simulink model "nn"  (R2018b)
settings: Solver=VariableStepAuto  StartTime=0.0  StopTime=10.0  RelTol=1e-3
libraries: neural x28
settings Model: Creator=Mihail  LastModifiedBy=Mihail

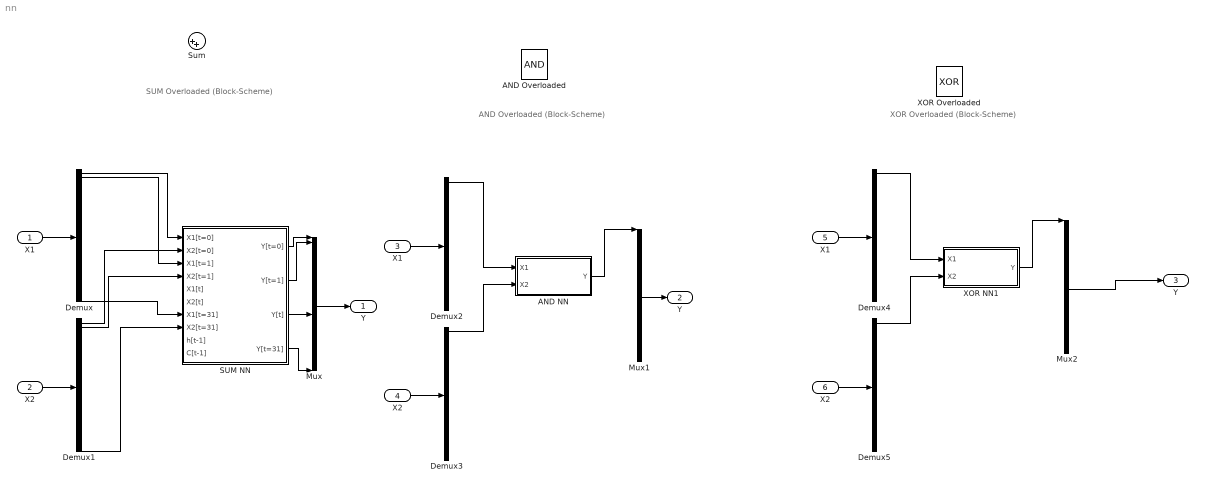
== system nn ==
  note: SUM Overloaded
      | (Block-Scheme)
  note: AND Overloaded
      | (Block-Scheme)
  note: XOR Overloaded
      | (Block-Scheme)
  X1 : Inport
  X2 : Inport  Port=2
  "X1 " : Inport  Port=3
  "X2 " : Inport  Port=4
  "X1   " : Inport  Port=5
  "X2  " : Inport  Port=6
  AND NN : Subsystem
  AND Overloaded : Logic  AllPortsSameDT=off  OutDataTypeStr=boolean
  Demux{,1..5} (6 alike) : Demux  Outputs=32
  Mux : Mux  Inputs=32
  Mux1 : Mux  Inputs=32
  Mux2 : Mux  Inputs=32
  SUM NN : Subsystem
  Sum : Sum  Inputs=|++
  XOR NN1 : Subsystem
  XOR Overloaded : Logic  Operator=XOR  AllPortsSameDT=off  OutDataTypeStr=boolean
  Y : Outport
  "Y " : Outport  Port=2
  "Y  " : Outport  Port=3
  wires:
  Demux/2 -> SUM NN/1(X1[t=0])
  Demux1/2 -> SUM NN/2(X2[t=0])
  Demux/3 -> SUM NN/3(X1[t=1])
  SUM NN/1(Y[t=0]) -> Mux/1
  SUM NN/2(Y[t=1]) -> Mux/2
  SUM NN/3(Y[t]) -> Mux/19
  SUM NN/4(Y[t=31]) -> Mux/32
  Demux/32 -> SUM NN/7(X1[t=31])
  Demux1/3 -> SUM NN/4(X2[t=1])
  Demux1/32 -> SUM NN/8(X2[t=31])
  X1/1 -> Demux/1
  X2/1 -> Demux1/1
  Mux/1 -> Y/1
  AND NN/1(Y) -> Mux1/1
  "X1 "/1 -> Demux2/1
  "X2 "/1 -> Demux3/1
  Demux2/2 -> AND NN/1(X1)
  Demux3/2 -> AND NN/2(X2)
  Mux1/1 -> "Y "/1
  Demux4/2 -> XOR NN1/1(X1)
  "X1   "/1 -> Demux4/1
  "X2  "/1 -> Demux5/1
  Demux5/2 -> XOR NN1/2(X2)
  XOR NN1/1(Y) -> Mux2/1
  Mux2/1 -> "Y  "/1

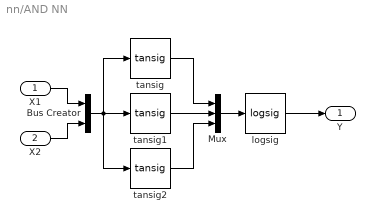
== system nn/AND NN ==
  X1 : Inport
  X2 : Inport  Port=2
  Bus Creator : BusCreator  Inputs=2
  Mux : Mux  Inputs=3
  logsig : neural/Transfer Functions/logsig
  tansig : neural/Transfer Functions/tansig
  tansig1 : neural/Transfer Functions/tansig
  tansig2 : neural/Transfer Functions/tansig
  Y : Outport
  wires:
  tansig2/1 -> Mux/3
  tansig1/1 -> Mux/2
  tansig/1 -> Mux/1
  Mux/1 -> logsig/1
  logsig/1 -> Y/1
  X1/1 -> Bus Creator/1
  X2/1 -> Bus Creator/2
  Bus Creator/1 -> tansig/1, tansig2/1, tansig1/1

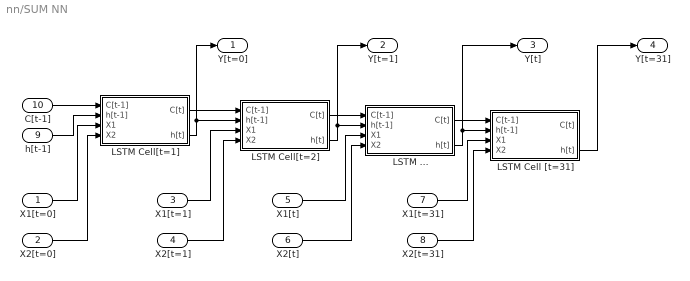
== system nn/SUM NN ==
  X1[t=0] : Inport
  X2[t=0] : Inport  Port=2
  X1[t=1] : Inport  Port=3
  X2[t=1] : Inport  Port=4
  X1[t] : Inport  Port=5
  X2[t] : Inport  Port=6
  X1[t=31] : Inport  Port=7
  X2[t=31] : Inport  Port=8
  h[t-1] : Inport  Port=9
  C[t-1] : Inport  Port=10
  LSTM ... : Subsystem
  LSTM Cell [t=31] : Subsystem
  LSTM Cell[t=1] : Subsystem
  LSTM Cell[t=2] : Subsystem
  Y[t=0] : Outport
  Y[t=1] : Outport  Port=2
  Y[t] : Outport  Port=3
  Y[t=31] : Outport  Port=4
  wires:
  C[t-1]/1 -> LSTM Cell[t=1]/1(C[t-1])
  h[t-1]/1 -> LSTM Cell[t=1]/2(h[t-1])
  LSTM Cell[t=1]/1(C[t]) -> LSTM Cell[t=2]/1(C[t-1])
  LSTM Cell[t=1]/2(h[t]) -> Y[t=0]/1, LSTM Cell[t=2]/2(h[t-1])
  X1[t=0]/1 -> LSTM Cell[t=1]/3(X1)
  X2[t=0]/1 -> LSTM Cell[t=1]/4(X2)
  X1[t=1]/1 -> LSTM Cell[t=2]/3(X1)
  X2[t=1]/1 -> LSTM Cell[t=2]/4(X2)
  LSTM Cell[t=2]/1(C[t]) -> LSTM .../1(C[t-1])
  LSTM Cell[t=2]/2(h[t]) -> Y[t=1]/1, LSTM .../2(h[t-1])
  LSTM .../1(C[t]) -> LSTM Cell [t=31]/1(C[t-1])
  X2[t]/1 -> LSTM .../4(X2)
  X1[t]/1 -> LSTM .../3(X1)
  X1[t=31]/1 -> LSTM Cell [t=31]/3(X1)
  X2[t=31]/1 -> LSTM Cell [t=31]/4(X2)
  LSTM Cell [t=31]/2(h[t]) -> Y[t=31]/1
  LSTM .../2(h[t]) -> Y[t]/1, LSTM Cell [t=31]/2(h[t-1])

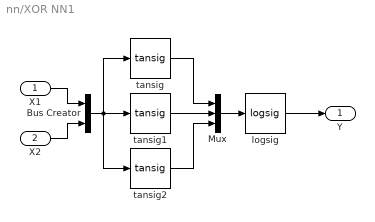
== system nn/XOR NN1 ==
  X1 : Inport
  X2 : Inport  Port=2
  Bus Creator : BusCreator  Inputs=2
  Mux : Mux  Inputs=3
  logsig : neural/Transfer Functions/logsig
  tansig : neural/Transfer Functions/tansig
  tansig1 : neural/Transfer Functions/tansig
  tansig2 : neural/Transfer Functions/tansig
  Y : Outport
  wires:
  tansig2/1 -> Mux/3
  tansig1/1 -> Mux/2
  tansig/1 -> Mux/1
  Mux/1 -> logsig/1
  logsig/1 -> Y/1
  X1/1 -> Bus Creator/1
  X2/1 -> Bus Creator/2
  Bus Creator/1 -> tansig/1, tansig2/1, tansig1/1

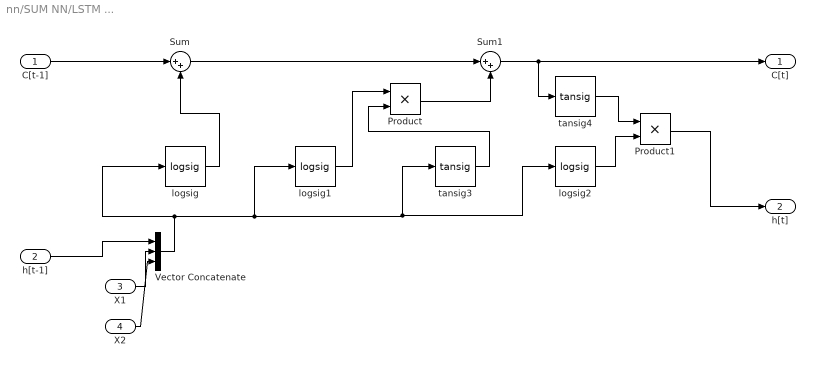
== system nn/SUM NN/LSTM ... ==
  C[t-1] : Inport
  h[t-1] : Inport  Port=2
  X1 : Inport  Port=3
  X2 : Inport  Port=4
  Product : Product
  Product1 : Product
  Sum : Sum  Inputs=|++
  Sum1 : Sum  Inputs=|++
  Vector Concatenate : Concatenate  NumInputs=3
  logsig : neural/Transfer Functions/logsig
  logsig1 : neural/Transfer Functions/logsig
  logsig2 : neural/Transfer Functions/logsig
  tansig3 : neural/Transfer Functions/tansig
  tansig4 : neural/Transfer Functions/tansig
  C[t] : Outport
  h[t] : Outport  Port=2
  wires:
  h[t-1]/1 -> Vector Concatenate/1
  X1/1 -> Vector Concatenate/2
  X2/1 -> Vector Concatenate/3
  Vector Concatenate/1 -> tansig3/1, logsig2/1, logsig1/1, logsig/1
  C[t-1]/1 -> Sum/1
  logsig/1 -> Sum/2
  Sum/1 -> Sum1/1
  tansig3/1 -> Product/2
  logsig1/1 -> Product/1
  Product/1 -> Sum1/2
  logsig2/1 -> Product1/2
  Sum1/1 -> C[t]/1, tansig4/1
  tansig4/1 -> Product1/1
  Product1/1 -> h[t]/1

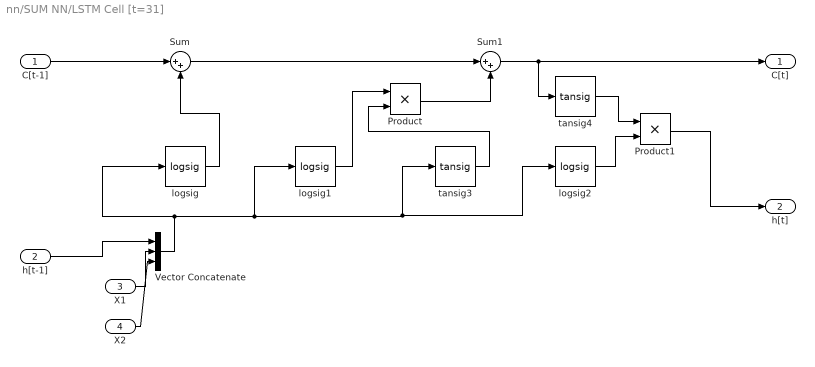
== system nn/SUM NN/LSTM Cell [t=31] ==
  C[t-1] : Inport
  h[t-1] : Inport  Port=2
  X1 : Inport  Port=3
  X2 : Inport  Port=4
  Product : Product
  Product1 : Product
  Sum : Sum  Inputs=|++
  Sum1 : Sum  Inputs=|++
  Vector Concatenate : Concatenate  NumInputs=3
  logsig : neural/Transfer Functions/logsig
  logsig1 : neural/Transfer Functions/logsig
  logsig2 : neural/Transfer Functions/logsig
  tansig3 : neural/Transfer Functions/tansig
  tansig4 : neural/Transfer Functions/tansig
  C[t] : Outport
  h[t] : Outport  Port=2
  wires:
  h[t-1]/1 -> Vector Concatenate/1
  X1/1 -> Vector Concatenate/2
  X2/1 -> Vector Concatenate/3
  Vector Concatenate/1 -> tansig3/1, logsig2/1, logsig1/1, logsig/1
  C[t-1]/1 -> Sum/1
  logsig/1 -> Sum/2
  Sum/1 -> Sum1/1
  tansig3/1 -> Product/2
  logsig1/1 -> Product/1
  Product/1 -> Sum1/2
  logsig2/1 -> Product1/2
  Sum1/1 -> C[t]/1, tansig4/1
  tansig4/1 -> Product1/1
  Product1/1 -> h[t]/1

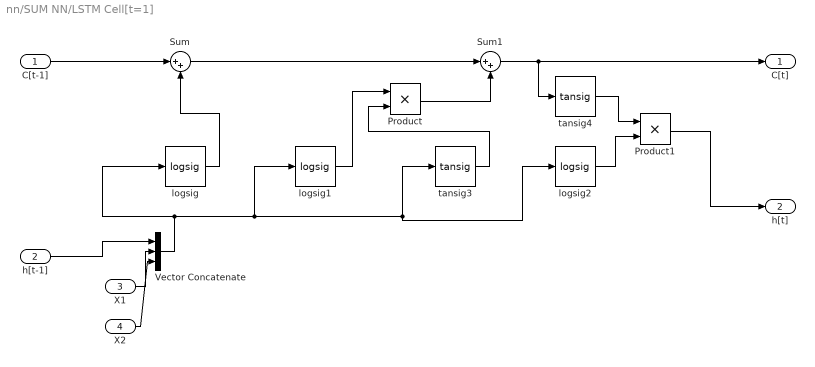
== system nn/SUM NN/LSTM Cell[t=1] ==
  C[t-1] : Inport
  h[t-1] : Inport  Port=2
  X1 : Inport  Port=3
  X2 : Inport  Port=4
  Product : Product
  Product1 : Product
  Sum : Sum  Inputs=|++
  Sum1 : Sum  Inputs=|++
  Vector Concatenate : Concatenate  NumInputs=3
  logsig : neural/Transfer Functions/logsig
  logsig1 : neural/Transfer Functions/logsig
  logsig2 : neural/Transfer Functions/logsig
  tansig3 : neural/Transfer Functions/tansig
  tansig4 : neural/Transfer Functions/tansig
  C[t] : Outport
  h[t] : Outport  Port=2
  wires:
  h[t-1]/1 -> Vector Concatenate/1
  X1/1 -> Vector Concatenate/2
  X2/1 -> Vector Concatenate/3
  Vector Concatenate/1 -> tansig3/1, logsig2/1, logsig1/1, logsig/1
  C[t-1]/1 -> Sum/1
  logsig/1 -> Sum/2
  Sum/1 -> Sum1/1
  tansig3/1 -> Product/2
  logsig1/1 -> Product/1
  Product/1 -> Sum1/2
  logsig2/1 -> Product1/2
  Sum1/1 -> C[t]/1, tansig4/1
  tansig4/1 -> Product1/1
  Product1/1 -> h[t]/1

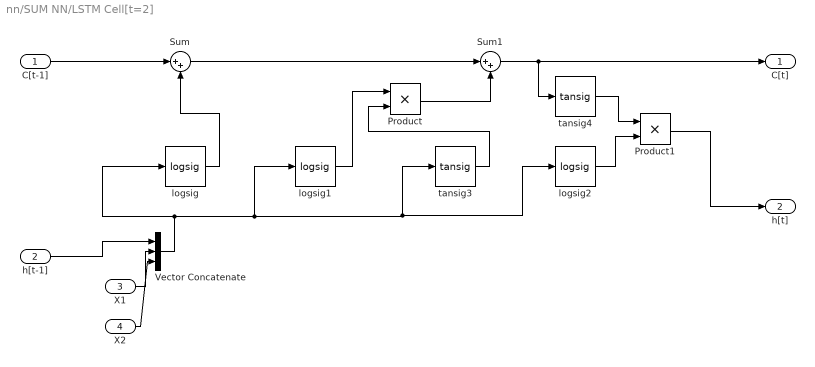
== system nn/SUM NN/LSTM Cell[t=2] ==
  C[t-1] : Inport
  h[t-1] : Inport  Port=2
  X1 : Inport  Port=3
  X2 : Inport  Port=4
  Product : Product
  Product1 : Product
  Sum : Sum  Inputs=|++
  Sum1 : Sum  Inputs=|++
  Vector Concatenate : Concatenate  NumInputs=3
  logsig : neural/Transfer Functions/logsig
  logsig1 : neural/Transfer Functions/logsig
  logsig2 : neural/Transfer Functions/logsig
  tansig3 : neural/Transfer Functions/tansig
  tansig4 : neural/Transfer Functions/tansig
  C[t] : Outport
  h[t] : Outport  Port=2
  wires:
  h[t-1]/1 -> Vector Concatenate/1
  X1/1 -> Vector Concatenate/2
  X2/1 -> Vector Concatenate/3
  Vector Concatenate/1 -> tansig3/1, logsig2/1, logsig1/1, logsig/1
  C[t-1]/1 -> Sum/1
  logsig/1 -> Sum/2
  Sum/1 -> Sum1/1
  tansig3/1 -> Product/2
  logsig1/1 -> Product/1
  Product/1 -> Sum1/2
  logsig2/1 -> Product1/2
  Sum1/1 -> C[t]/1, tansig4/1
  tansig4/1 -> Product1/1
  Product1/1 -> h[t]/1
